simulink model "targetFile0"  (R2018a)
settings: Solver=VariableStepAuto  StartTime=0.0  StopTime=10.0  RelTol=1e-3
settings Model: Creator=PC_393_ADMIN  LastModifiedBy=PC_393_ADMIN

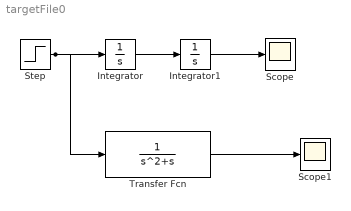
== system targetFile0 ==
  Integrator : Integrator
  Integrator1 : Integrator
  Scope : Scope
  Scope1 : Scope
  Step : Step  SampleTime=0
  Transfer Fcn : TransferFcn  Denominator=[1 1 0]
  wires:
  Step/1 -> Integrator/1, Transfer Fcn/1
  Integrator/1 -> Integrator1/1
  Integrator1/1 -> Scope/1
  Transfer Fcn/1 -> Scope1/1
